simulink model "motore_PI"  (R2022a)
settings: Solver=ode45  StartTime=0.0  StopTime=5  MaxStep=0.001  RelTol=1e-3
values from neighbouring files (symbols this model uses):
  d = 1 / sqrt(2)    [ex1.m]    (also in ex2.m)
  Kp = kc / 4    [ex2.m]    (also in ex3.m = 0.7442)
  w = step(Ww, t, w1)    [ex2.m]
  w0 = 0    [ex3.m]
undefined symbols (not defined in the file or in its folder): diff, mot
settings Model: Creator=loren  LastModifiedBy=loren
settings DataIOCC: ReturnWorkspaceOutputs=off

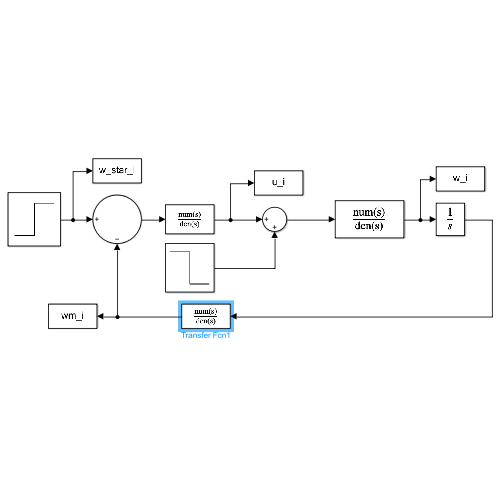
[thumbnail: Simulink's stored preview of the top-level diagram]
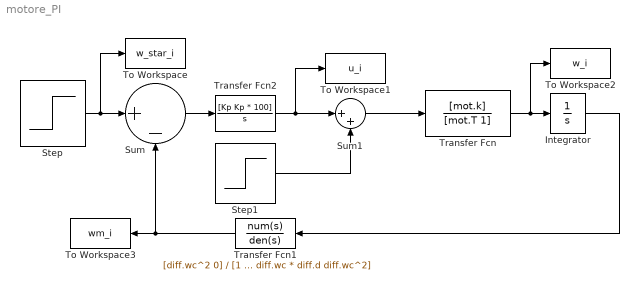
== system motore_PI ==
  Integrator : Integrator  InitialCondition=w0
  Step : Step  Time=w.t  After=w.A  SampleTime=0
  Step1 : Step  Time=d.t  After=d.A  SampleTime=0
  Sum : Sum  Inputs=|+-
  Sum1 : Sum  Inputs=|++
  To Workspace : ToWorkspace  VariableName=w_star_i  SaveFormat=Timeseries  SampleTime=-1
  To Workspace1 : ToWorkspace  VariableName=u_i  SaveFormat=Timeseries  SampleTime=-1
  To Workspace2 : ToWorkspace  VariableName=w_i  SaveFormat=Timeseries  SampleTime=-1
  To Workspace3 : ToWorkspace  VariableName=wm_i  SaveFormat=Timeseries  SampleTime=-1
  Transfer Fcn : TransferFcn  Numerator=[mot.k]  Denominator=[mot.T 1]
  Transfer Fcn1 : TransferFcn  Numerator=[diff.wc^2 0]  Denominator=[1 2 * diff.wc * diff.d diff.wc^2]
  Transfer Fcn2 : TransferFcn  Numerator=[Kp Kp * 100]  Denominator=[1 0]
  wires:
  Step1/1 -> Sum1/2
  Integrator/1 -> Transfer Fcn1/1
  Sum/1 -> Transfer Fcn2/1
  Step/1 -> Sum/1, To Workspace/1
  Sum1/1 -> Transfer Fcn/1
  Transfer Fcn1/1 -> Sum/2, To Workspace3/1
  Transfer Fcn2/1 -> Sum1/1, To Workspace1/1
  Transfer Fcn/1 -> Integrator/1, To Workspace2/1
